simulink model "model_sim_fuzzy"  (R2024b)
settings: Solver=FixedStepAuto  StartTime=0.0  StopTime=tsim  FixedStep=T  RelTol=1e-3
undefined symbols (not defined in the file or in its folder): C0, C1, Cd, Ce
libraries: fuzblock x2
settings Model: Creator=usuario  LastModifiedBy=usuario
settings DataIOCC: ReturnWorkspaceOutputs=off  TimeSaveName=t
settings RTWCC: GPUComputeCapability=3.5

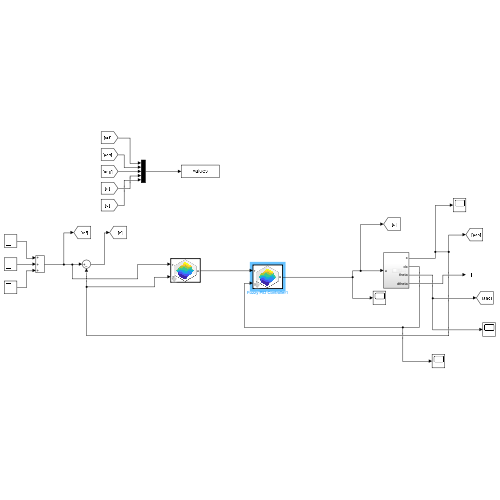
[thumbnail: Simulink's stored preview of the top-level diagram]
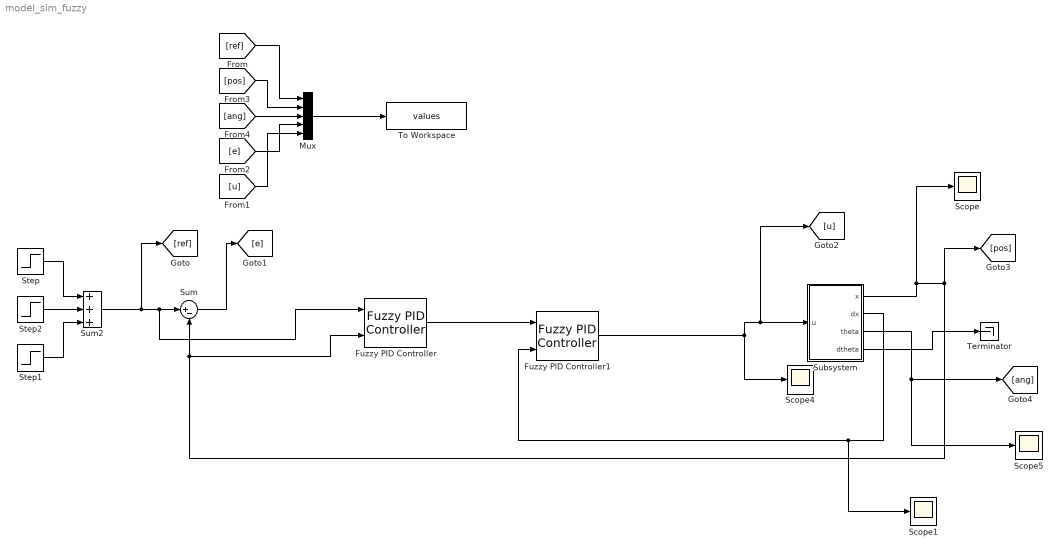
== system model_sim_fuzzy ==
  Fuzzy PID Controller : fuzblock/Fuzzy PID Controller  TimeDomainType=Discrete-time  CE=Ce(1)  CD=Cd(1)  C0=C0(1)  C1=C1(1)  UseAccumulator=off  IntegratorMethod=Trapezoidal  DerivativeSignal=Process output (y)  UseFilter=on  N=100  DerivativeFilterMethod=Trapezoidal  AddFFRefIn=on  E=off  SampleTime=-1  FIS="\"PID.fis\""  OutputSampleNumber=101  UseLookupTable=on  NumBreakpoints=100
  Fuzzy PID Controller1 : fuzblock/Fuzzy PID Controller  TimeDomainType=Discrete-time  CE=Ce(2)  CD=Cd(2)  C0=C0(2)  C1=C1(2)  UseAccumulator=off  IntegratorMethod=Trapezoidal  DerivativeSignal=Process output (y)  UseFilter=on  N=100  DerivativeFilterMethod=Trapezoidal  AddFFRefIn=on  E=off  SampleTime=-1  FIS="\"PID.fis\""  OutputSampleNumber=101  UseLookupTable=on  NumBreakpoints=100
  Mux : Mux  Inputs=5
  Scope{,1,4..5} (4 alike) : Scope
  Step : Step  Time=0  After=0.6  SampleTime=0
  Step1 : Step  Time=30  After=-0.7  SampleTime=0
  Step2 : Step  Time=15  After=0.4  SampleTime=0
  Subsystem : Subsystem
  Sum : Sum  Inputs=|+-
  Sum2 : Sum  Inputs=+++
  Terminator : Terminator
  To Workspace : ToWorkspace  VariableName=values  SaveFormat=Structure  SampleTime=-1
  wires:
  Mux/1 -> To Workspace/1
  Subsystem/1(x) -> Scope/1, Fuzzy PID Controller/2, Sum/2, [pos]
  Subsystem/3(theta) -> [ang], Scope5/1
  Sum2/1 -> [ref], Fuzzy PID Controller/1, Sum/1
  Subsystem/4(dtheta) -> Terminator/1
  [ref] -> Mux/1
  [pos] -> Mux/2
  [ang] -> Mux/3
  [e] -> Mux/4
  [u] -> Mux/5
  Sum/1 -> [e]
  Step/1 -> Sum2/1
  Step1/1 -> Sum2/3
  Step2/1 -> Sum2/2
  Subsystem/2(dx) -> Scope1/1, Fuzzy PID Controller1/2
  Fuzzy PID Controller/1 -> Fuzzy PID Controller1/1
  Fuzzy PID Controller1/1 -> [u], Subsystem/1(u), Scope4/1

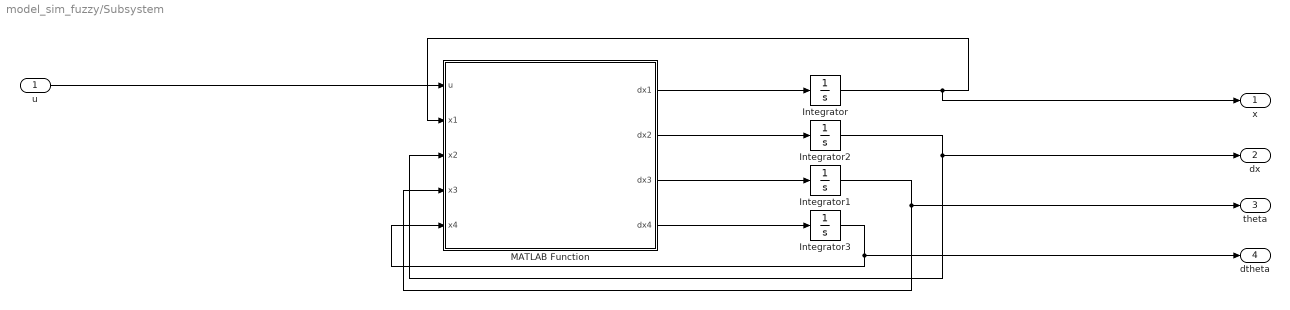
== system model_sim_fuzzy/Subsystem ==
  u : Inport
  Integrator : Integrator  InitialCondition=0.002
  Integrator1 : Integrator  InitialCondition=0.001
  Integrator2 : Integrator
  Integrator3 : Integrator
  MATLAB Function : MATLAB Function  TreatAsAtomicUnit=on
  x : Outport
  dx : Outport  Port=2
  theta : Outport  Port=3
  dtheta : Outport  Port=4
  wires:
  MATLAB Function/2(dx2) -> Integrator2/1
  Integrator/1 -> x/1, MATLAB Function/2(x1)
  Integrator2/1 -> MATLAB Function/3(x2), dx/1
  MATLAB Function/4(dx4) -> Integrator3/1
  MATLAB Function/1(dx1) -> Integrator/1
  MATLAB Function/3(dx3) -> Integrator1/1
  Integrator3/1 -> MATLAB Function/5(x4), dtheta/1
  Integrator1/1 -> theta/1, MATLAB Function/4(x3)
  u/1 -> MATLAB Function/1(u)

== matlab function model_sim_fuzzy/Subsystem/MATLAB Function ==
  data: u input; dx1 output; x1 input; x2 input; x3 input; x4 input; dx2 output; dx3 output; dx4 output
function [dx1,dx2,dx3,dx4] = plant_model(u,x1,x2,x3,x4)
M = 10;g=9.8;m=0.8;l=0.5;mu=0.05;
q = [x1;x2;x3;x4];
a11 = -mu/(M+m*sin(x3)^2); a12 = m*g*cos(x3)*sin(x3)/((M+m*sin(x3)^2)*x3);
a13 = m*l*x4*sin(x3)/(M+m*sin(x3)^2); a21 = mu*cos(x3)/(l*(M+m*sin(x3)^2));
a22 = -(M+m)*g*sin(x3)/(l*x3*(M+m*sin(x3)^2)); a23=-m*x4*sin(x3)*cos(x3)/(M+m*sin(x3)^2);
b1 = 1/(M+m*sin(x3)^2); b2 = -cos(x3)/(l*(M+m*sin(x3)^2));
A = [0 1 0 0;0 a11 a12 a13;0 0 0 1;0 a21 a22 a23];
B = [0;b1;0;b2];

dq = A*q + B*u;
dx1 = dq(1);
dx2 = dq(2);
dx3 = dq(3);
dx4 = dq(4);
